simulink model "Grades"  (R2018b)
settings: Solver=FixedStepDiscrete  StartTime=0.0  StopTime=10.0  RelTol=1e-3
settings Model: Creator=Ahmed Soliman  LastModifiedBy=Ahmed Soliman
settings OptimizationCC: DefaultParameterBehavior=Inlined  EnhancedBackFolding=on  PassReuseOutputArgsAs=Individual arguments  OptimizeBlockOrder=speed  DifferentSizesBufferReuse=on  OptimizationCustomize=off
settings DebuggingCC: UnderspecifiedInitializationDetection=Classic  MergeDetectMultiDrivingBlocksExec=none  ParameterTunabilityLossMsg=error
settings ModelReferenceCC: PropagateSignalLabelsOutOfModel=off
settings SFSimCC: MATLABDynamicMemAlloc=off
settings RTWCC: SystemTargetFile=ert.tlc  GenCodeOnly=on  TemplateMakefile=ert_default_tmf  GenerateReport=on  IncludeHyperlinkInReport=on  LaunchReport=on  GenerateTraceInfo=on  GenerateTraceReport=on  GenerateTraceReportSl=on  GenerateTraceReportSf=on  GenerateTraceReportEml=on
settings CodeAppCC: ForceParamTrailComments=on  IgnoreCustomStorageClasses=off  OperatorAnnotations=on  SimulinkDataObjDesc=on  SFDataObjDesc=on  InsertBlockDesc=on
settings ERTTargetCC: TargetLangStandard=C99 (ISO)  GenerateSampleERTMain=on  InlinedParameterPlacement=NonHierarchical  ERTCustomFileTemplate=example_file_process.tlc

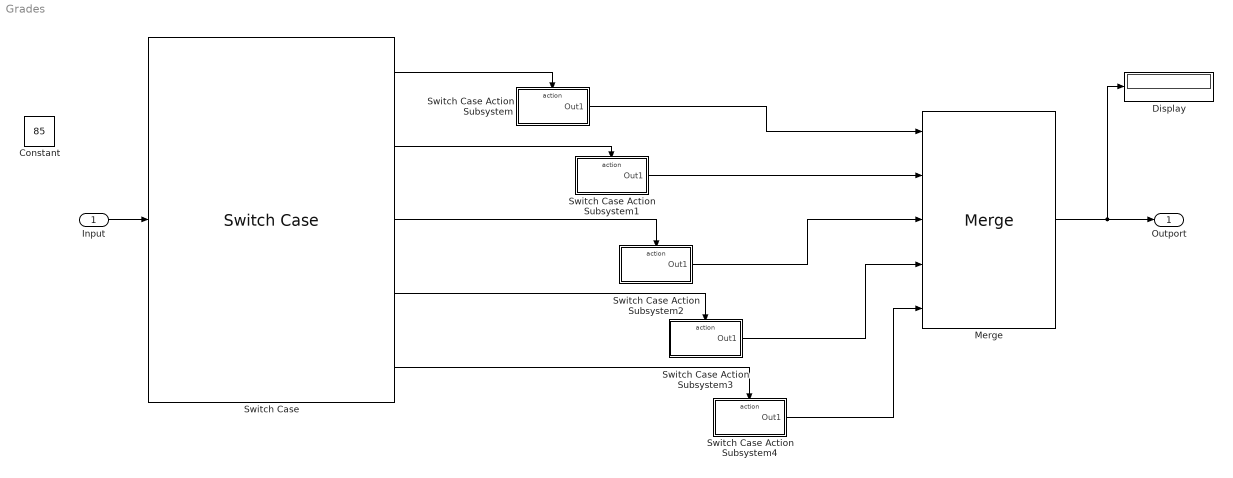
== system Grades ==
  Input : Inport  OutDataTypeStr=uint32
  Constant : Constant  Value=85
  Display : Display
  Merge : Merge  Inputs=5
  Switch Case : SwitchCase  CaseConditions={85:100,75:84,65:74,55:64}
  Switch Case Action Subsystem : Subsystem  TreatAsAtomicUnit=on
  Switch Case Action Subsystem1 : Subsystem  TreatAsAtomicUnit=on
  Switch Case Action Subsystem2 : Subsystem  TreatAsAtomicUnit=on
  Switch Case Action Subsystem3 : Subsystem  TreatAsAtomicUnit=on
  Switch Case Action Subsystem4 : Subsystem  TreatAsAtomicUnit=on
  Outport : Outport
  wires:
  Switch Case/1 -> Switch Case Action Subsystem/Action
  Switch Case/2 -> Switch Case Action Subsystem1/Action
  Switch Case/3 -> Switch Case Action Subsystem2/Action
  Switch Case/4 -> Switch Case Action Subsystem3/Action
  Switch Case/5 -> Switch Case Action Subsystem4/Action
  Switch Case Action Subsystem/1(Out1) -> Merge/1
  Switch Case Action Subsystem1/1(Out1) -> Merge/2
  Switch Case Action Subsystem2/1(Out1) -> Merge/3
  Switch Case Action Subsystem3/1(Out1) -> Merge/4
  Switch Case Action Subsystem4/1(Out1) -> Merge/5
  Merge/1 -> Display/1, Outport/1
  Input/1 -> Switch Case/1

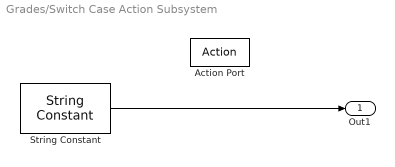
== system Grades/Switch Case Action Subsystem ==
  Action Port : ActionPort  ActionType=case
  String Constant : StringConstant  String="\"A\""
  Out1 : Outport
  wires:
  String Constant/1 -> Out1/1

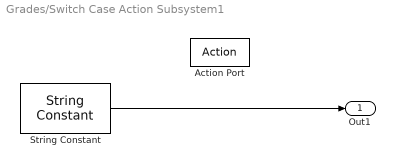
== system Grades/Switch Case Action Subsystem1 ==
  Action Port : ActionPort  ActionType=case
  String Constant : StringConstant  String="\"B\""
  Out1 : Outport
  wires:
  String Constant/1 -> Out1/1

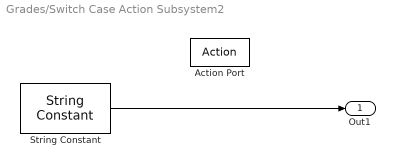
== system Grades/Switch Case Action Subsystem2 ==
  Action Port : ActionPort  ActionType=case
  String Constant : StringConstant  String="\"C\""
  Out1 : Outport
  wires:
  String Constant/1 -> Out1/1

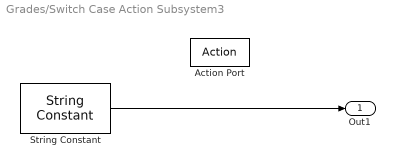
== system Grades/Switch Case Action Subsystem3 ==
  Action Port : ActionPort  ActionType=case
  String Constant : StringConstant  String="\"D\""
  Out1 : Outport
  wires:
  String Constant/1 -> Out1/1

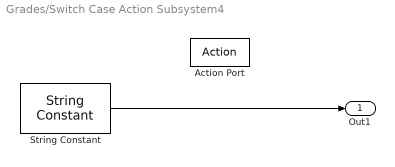
== system Grades/Switch Case Action Subsystem4 ==
  Action Port : ActionPort  ActionType=default
  String Constant : StringConstant  String="\"F\""
  Out1 : Outport
  wires:
  String Constant/1 -> Out1/1
